simulink model "apilot2"  (Simulink 2.09)
settings: Solver=ode15s  StartTime=0.0  StopTime=140  MaxStep=4  RelTol=1e-04  AbsTol=1e-04
values from neighbouring files (symbols this model uses):
  CD = 0    [apinit.m]    (also in vorinit.m)
  gamgs = -3*pi/180    (= -0.0523598775598)    [apinit.m]    (also in ilsinit.m = -3)
  HRW = 0    [apinit.m]    (also in ilsinit.m)
  Sgs = 625/abs(gamgs)    [apinit.m]    (also in ilsinit.m)
  Sloc = 1.4*xloc    (= 2800)    [apinit.m]    (also in ilsinit.m)
  xgs = 300    [apinit.m]    (also in ilsinit.m)
  xloc = 2000    [apinit.m]    (also in ilsinit.m)
  ymod1A = [1 1 1 0 0]'    [apmode.m]
  ymod1S = [1 1 1 0 0]'    [apmode.m]
  ymod2A = [1 1 0 0 1]'    [apmode.m]
  ymod2S = [1 1 0 0 1]'    [apmode.m]
  yrefA = [0 Dpsir]'    [apmode.m]
  yrefS = [0 0 DHdotr]'    [apmode.m]
undefined symbols (not defined in the file or in its folder): Aail, Aelv, AM, Arud, Bail, Belv, Brud, Cail, Celv, Crud, Dail, Delv, Drud, GM1, sfunyst, uaero0, uprop0, xdot0, xfix, xinco
libraries: navlib1 x1, navlib2 x1
(part 1 of 2)
settings Model: SaveTime=off  SaveOutput=off  ConsistencyChecking=off  RTWTemplateMakefile=grt_vc.tmf

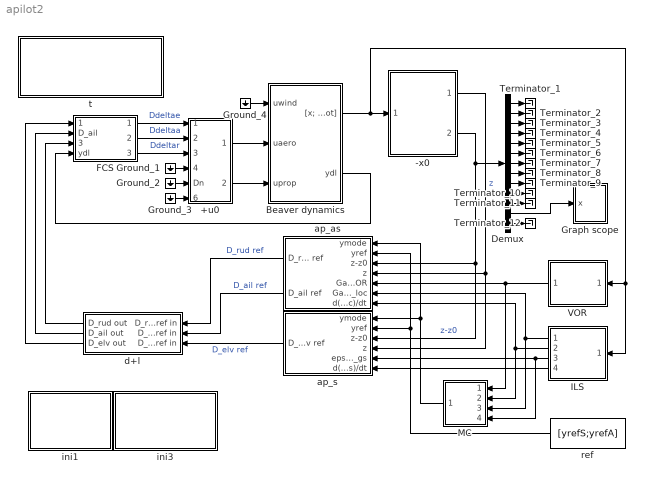
== system apilot2 ==
  +u0 : Subsystem
      mask Display: disp('Add\ninitial\ninputs')
  -x0 : Subsystem
      mask Display: disp('Subtract\ninitial con-\nditions\n\nNo sensors!')
  Beaver dynamics : Subsystem
  Demux : Demux  Outputs=13
  FCS : Subsystem
      mask Display: disp('Actuator &\ncable dy-\nnamics')
  Graph scope : Subsystem  mask(Storage scope.){npts=100, color='g-'}
      mask prompts: npts "Initial Time Range:"; color "Initial y-min:"
      mask help:
      | Storage scope using MATLAB graph window.
      | Enter plotting ranges and line type.
      mask init:
      | close all; ax = [0, @1, @2, @3];
      mask Help: Uses MATLAB's graph window.\nUse only one block per system.\nLine type must be in quotes.\nSee the M-file sfunyst.m.
      mask Display: plot(0,0,100,100,[83,76,63,52,42,38,28,16,11,84,11,11,11,90,90,11],[75,58,47,54,72,80,84,74,65,65,65,90,40,40,90,90])
  Ground_{1..4} (4 alike) : Ground
  ILS : Subsystem  Orientation=left
      mask Display: plot(0,0,100,100,[53,23,30,61,53],[45,60,64,49,45],[16,27,32,26],[48,40,43,47],[21,20,24,26,21],[44,55,56,47,44],[20,20,16],[50,50,48],[38,27,26,33],[52,46,48,55],[42,38,27],[50,47,46],[40,44,44,45,45,44,42],[48,44,42,42,44,44,50],[47,45,43],[55,58,58],[54,84,98,90,54],[36,21,56,58,36],[74,68],[34,29],[81,76],[43,38],[87,83],[49,45],[94,89],[57,52],[105,105],[0,0])
  MC : Subsystem  Orientation=left
      mask Display: disp('Mode\nCon-\ntroller')
  Terminator_{1..12} (12 alike) : Terminator
  VOR : Subsystem  Orientation=left
      mask Display: plot(0,0,100,100,[86,85,90,86,80,85,0],[16,80,20,16,20,80,62],[22,18,25,28,22,19],[36,32,29,33,36,45],[17,15,12,18,16,19],[37,37,34,32,44,46],[22,31,47,52,19,15,28,22],[36,44,39,44,55,50,45,38],[31,28],[44,45],[20,18,17],[31,30,32],[36,35,36,37,36,35,35,35,33,31,25],[41,38,33,32,30,30,32,33,37,35,34],[85,42],[80,50],[86,87,87,86,84,83,84,85],[83,81,78,76,76,79,82,83])
  ap_as : Subsystem  Orientation=left
      mask Display: disp('Asymmetrical\nautopilot\nmodes')
  ap_s : Subsystem  Orientation=left
      mask Display: disp('Symmetrical\nautopilot\nmodes')
  d+l : Subsystem  Orientation=left
      mask Display: disp('computational\ndelay & limiters')
  ini1 : Subsystem
      settings: OpenFcn=apinit
      mask Type: apinit
      mask Display: disp('1. Initialize\nsubsystems\n\nAPINIT')
  ini3 : Subsystem
      settings: OpenFcn=apmode
      mask Type: apmode
      mask Display: disp('2. Select mode &\nreference signals\n\nAPMODE')
  ref : Constant  Orientation=left  Value=[yrefS;yrefA]
      mask Display: disp('Reference\nsignals')
  t : Subsystem
      settings: OpenFcn=fdchelp apilot
      mask Display: disp('Apilot2 (no wind, turbu-\nlence, and sensor models,\nno ILS/VOR error signals)\nMarc Rauw, June 2000')
  wires:
  FCS/1(Ddeltae) -> +u0/1(Ddeltae)  "Ddeltae"
  FCS/2(Ddeltaa) -> +u0/2(Ddeltaa)  "Ddeltaa"
  FCS/3(Ddeltar) -> +u0/3(Ddeltar)  "Ddeltar"
  Ground_1/1 -> +u0/4(Ddeltaf)
  Ground_2/1 -> +u0/5(Dn)
  Ground_3/1 -> +u0/6(Dpz)
  Demux/12 -> Graph scope/1(x)
  ILS/2(d(Gamma_loc)/dt) -> ap_as/7(d(Gamma_loc)/dt), MC/2(d(Gamma_loc)/dt)
  -x0/2(z-z0 == [x-x0; Hdot-Hdot0]) -> Demux/1, ap_s/3(z-z0), ap_as/3(z-z0)  "z-z0"
  d+l/1(D_rud out) -> FCS/3(D_rud)
  d+l/2(D_ail out) -> FCS/2(D_ail)
  Beaver dynamics/1("[x; Hdot]") -> VOR/1("[x' ; Hdot]'"), ILS/1("[x' ;Hdot]'"), -x0/1("[x; Hdot]")
  Beaver dynamics/2(ydl) -> FCS/4(ydl)
  ap_as/2(D_ail ref) -> d+l/2(D_ail ref in)  "D_ail ref"
  ap_s/1(D_elv ref) -> d+l/3(D_elv ref in)  "D_elv ref"
  d+l/3(D_elv out) -> FCS/1(D_elv)
  ref/1 -> ap_s/2(yref), ap_as/2(yref)
  MC/1(ymode) -> ap_s/1(ymode), ap_as/1(ymode)
  +u0/1(uaero) -> Beaver dynamics/2(uaero)
  -x0/1("z == [x; Hdot] ") -> ap_as/4(z), ap_s/4(z)  "z"
  +u0/2(uprop) -> Beaver dynamics/3(uprop)
  VOR/1(Gamma_VOR) -> MC/1(Gamma_VOR), ap_as/5(Gamma_VOR)
  ILS/4(d(epsilon_gs)/dt) -> ap_s/6(d(epsilon_gs)/dt)
  ILS/1(Gamma_loc) -> MC/3(Gamma_loc), ap_as/6(Gamma_loc)
  ap_as/1(D_rud ref) -> d+l/1(D_rud ref in)  "D_rud ref"
  ILS/3(epsilon_gs) -> MC/4(epsilon_gs), ap_s/5(epsilon_gs)
  Demux/1 -> Terminator_1/1
  Demux/2 -> Terminator_2/1
  Demux/3 -> Terminator_3/1
  Demux/4 -> Terminator_4/1
  Demux/5 -> Terminator_5/1
  Demux/6 -> Terminator_6/1
  Demux/7 -> Terminator_7/1
  Demux/8 -> Terminator_8/1
  Demux/9 -> Terminator_9/1
  Demux/10 -> Terminator_10/1
  Demux/11 -> Terminator_11/1
  Demux/13 -> Terminator_12/1
  Ground_4/1 -> Beaver dynamics/1(uwind)

== system apilot2/+u0 ==
  note: Add initial inputs
  note: ENGINE INPUTS:
  note: AERODYNAMIC INPUTS:
  Ddeltae : Inport  Port=1  PortWidth=-1  SampleTime=-1
  Ddeltaa : Inport  Port=2  PortWidth=-1  SampleTime=-1
  Ddeltar : Inport  Port=3  PortWidth=-1  SampleTime=-1
  Ddeltaf : Inport  Port=4  PortWidth=-1  SampleTime=-1
  Dn : Inport  Port=5  PortWidth=-1  SampleTime=-1
  Dpz : Inport  Port=6  PortWidth=-1  SampleTime=-1
  Initial inputs for aeromod : Constant  Value=uaero0
  Initial inputs for engmod : Constant  Value=uprop0
  Mux1 : Mux  Inputs=4
  Mux2 : Mux  Inputs=2
  Sum : Sum  Inputs=++
  Sum1 : Sum  Inputs=++
  uaero : Outport  Port=1  InitialOutput=0
  uprop : Outport  Port=2  InitialOutput=0
  wires:
  Dpz/1 -> Mux2/2
  Dn/1 -> Mux2/1
  Initial inputs for engmod/1 -> Sum/2
  Mux2/1 -> Sum/1
  Sum/1 -> uprop/1
  Ddeltaa/1 -> Mux1/2
  Ddeltae/1 -> Mux1/1
  Ddeltar/1 -> Mux1/3
  Ddeltaf/1 -> Mux1/4
  Initial inputs for aeromod/1 -> Sum1/1
  Sum1/1 -> uaero/1
  Mux1/1 -> Sum1/2

== system apilot2/-x0 ==
  note: Subtract initial conditions
  "[x; Hdot]" : Inport  Port=1  PortWidth=-1  SampleTime=-1
  Initial condition : Constant  Value=[xinco; xdot0(12)]
  Sum : Sum  Inputs=+-
  "z == [x; Hdot] " : Outport  Port=1  InitialOutput=0
  z-z0 == [x-x0; Hdot-Hdot0] : Outport  Port=2  InitialOutput=0
  wires:
  "[x; Hdot]"/1 -> "z == [x; Hdot] "/1, Sum/1
  Initial condition/1 -> Sum/2
  Sum/1 -> z-z0 == [x-x0; Hdot-Hdot0]/1

== system apilot2/Beaver dynamics ==
  note: Beaver dynamics
      | and output equations
  uwind : Inport  Port=1  PortWidth=6  SampleTime=-1
  uaero : Inport  Port=2  PortWidth=4  SampleTime=-1
  uprop : Inport  Port=3  PortWidth=2  SampleTime=-1
  0 : Subsystem
      settings: OpenFcn=fdchelp level1
      mask Display: disp('Subsystem equivalent of\nthe S-function BEAVER\nM.O. Rauw, October 1997')
  AC : Subsystem
  Clock : Clock
  Demux1 : Demux  Outputs=[11 1]
  Mux : Mux  Inputs=[12 1]
  Mux_in : Mux  Orientation=up  Inputs=[4 2 6]
      settings: OpenFcn=fdchelp inputs
      mask Display: disp('Mux\nclick\n2x for\ninfo!')
  Mux_out : Mux  Orientation=up  Inputs=[12 12 3 3 3 4 2 6 6 6 6 6 3 3 5 3 3 3]
      settings: OpenFcn=fdchelp outputs
      mask Display: disp('Mux\n\nDouble-click for info!')
  Terminator_1 : Terminator
  To Workspace : ToWorkspace  VariableName=Out  SampleTime=0
      settings: Orientation=up  Buffer=5000
  "To Workspace " : ToWorkspace  VariableName=In  SampleTime=0
      settings: Orientation=up  Buffer=5000
  "To Workspace  " : ToWorkspace  VariableName=time  SampleTime=0
      settings: Buffer=5000
  "[x; Hdot]" : Outport  Port=1  InitialOutput=0
  ydl : Outport  Port=2  InitialOutput=0
  wires:
  Mux/1 -> "[x; Hdot]"/1
  Demux1/2 -> Mux/2  "Hdot"
  Demux1/1 -> Terminator_1/1
  uaero/1 -> Mux_in/1, AC/1(uaero)
  uprop/1 -> Mux_in/2, AC/2(uprop)
  uwind/1 -> Mux_in/3, AC/3(" uwind")
  AC/18(yad3) -> Mux_out/18
  AC/17(yad2) -> Mux_out/17
  AC/4(yuvw) -> Mux_out/4
  AC/1(x) -> Mux_out/1, Mux/1  "x"
  AC/3(ybvel) -> Mux_out/3
  AC/16(yad1) -> Mux_out/16
  AC/5(ydl) -> Mux_out/5, ydl/1
  AC/6(yfp) -> Mux_out/6
  AC/8(yacc) -> Mux_out/8
  AC/9(Caero) -> Mux_out/9
  AC/10(Cprop) -> Mux_out/10
  AC/11(FMaero) -> Mux_out/11
  AC/12(FMprop) -> Mux_out/12
  AC/13(Fgrav) -> Mux_out/13
  AC/14(Fwind) -> Mux_out/14
  AC/15(yatm) -> Mux_out/15
  AC/2(xdot) -> Demux1/1, Mux_out/2  "xdot"
  Clock/1 -> "To Workspace  "/1
  Mux_out/1 -> To Workspace/1
  Mux_in/1 -> "To Workspace "/1
  AC/7(ypow) -> Mux_out/7

== system apilot2/FCS ==
  note: Actuators
      | + cables:
  D_elv : Inport  Port=1  PortWidth=-1  SampleTime=-1
  D_ail : Inport  Port=2  PortWidth=-1  SampleTime=-1
  D_rud : Inport  Port=3  PortWidth=-1  SampleTime=-1
  ydl : Inport  Port=4  PortWidth=-1  SampleTime=-1
  Demux1 : Demux  Outputs=3
  Mux1 : Mux  Inputs=2
  Mux2 : Mux  Inputs=2
  Mux3 : Mux  Inputs=2
  ailerons : StateSpace  A=Aail  B=Bail  C=Cail*2  D=Dail  X0=0
  elevator : StateSpace  A=Aelv  B=Belv  C=Celv  D=Delv  X0=0
  rudder : StateSpace  A=Arud  B=Brud  C=Crud  D=Drud  X0=0
  t : Subsystem
      settings: OpenFcn=fdchelp actuatr
      mask Display: disp('Actuator & cable dynamics\nMarc Rauw, October 1997')
  Ddeltae : Outport  Port=1  InitialOutput=0
  Ddeltaa : Outport  Port=2  InitialOutput=0
  Ddeltar : Outport  Port=3  InitialOutput=0
  wires:
  Demux1/2 -> Mux1/2
  Demux1/1 -> Mux2/2
  Demux1/3 -> Mux3/2
  Mux1/1 -> elevator/1
  Mux2/1 -> ailerons/1
  Mux3/1 -> rudder/1
  elevator/1 -> Ddeltae/1
  ailerons/1 -> Ddeltaa/1
  ydl/1 -> Demux1/1
  rudder/1 -> Ddeltar/1
  D_elv/1 -> Mux1/1
  D_ail/1 -> Mux2/1
  D_rud/1 -> Mux3/1

== system apilot2/Graph scope ==
  x : Inport  Port=1  PortWidth=-1  SampleTime=-1
  "S-function M-file which plots lines " : S-Function  LoadFcn=sfunyst([],[],[],'LoadBlock')  FunctionName=sfunyst  Parameters=ax, color, npts
      settings: CopyFcn=sfunyst([],[],[],'CopyBlock')  DeleteFcn=sfunyst([],[],[],'DeleteBlock')
  wires:
  x/1 -> "S-function M-file which plots lines "/1

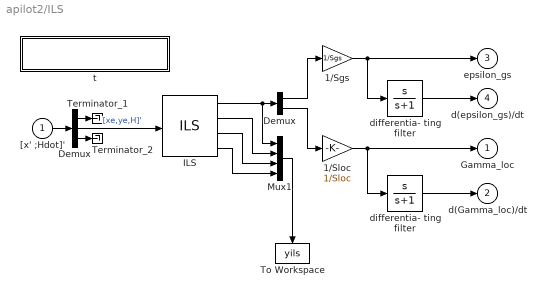
== system apilot2/ILS ==
  "[x' ;Hdot]'" : Inport  Port=1  PortWidth=-1  SampleTime=-1
  1/Sgs : Gain  Gain=1/Sgs
  1/Sloc : Gain  Gain=1/Sloc
  Demux : Demux  Outputs=2
  "Demux " : Demux  Outputs=[9 3 1]
  ILS : navlib1/ILS  RWpos=[20000,-100,0]  MaskParam1=0  MaskParam3=2200  MaskParam4=300  MaskParam5=100  MaskParam6=3
  Mux1 : Mux  Inputs=[2 2 6 2]
  Terminator_1 : Terminator
  Terminator_2 : Terminator
  To Workspace : ToWorkspace  VariableName=yils  SampleTime=0
      settings: Orientation=down  Buffer=5000
  differentia- ting filter : TransferFcn  Numerator=[1 0]  Denominator=[1 1]
  "differentia- ting filter " : TransferFcn  Numerator=[1 0]  Denominator=[1 1]
  t : Subsystem
      mask Display: disp('ILS signals (no error signals)\nMarc Rauw, January 1998')
  Gamma_loc : Outport  Port=1  InitialOutput=0
  d(Gamma_loc)/dt : Outport  Port=2  InitialOutput=0
  epsilon_gs : Outport  Port=3  InitialOutput=0
  d(epsilon_gs)/dt : Outport  Port=4  InitialOutput=0
  wires:
  Demux/2 -> 1/Sloc/1
  Demux/1 -> 1/Sgs/1
  ILS/2 -> Mux1/2
  ILS/3 -> Mux1/3
  ILS/1 -> Mux1/1, Demux/1
  ILS/4 -> Mux1/4
  Mux1/1 -> To Workspace/1
  1/Sloc/1 -> differentia- ting filter/1, Gamma_loc/1
  1/Sgs/1 -> "differentia- ting filter "/1, epsilon_gs/1
  differentia- ting filter/1 -> d(Gamma_loc)/dt/1
  "differentia- ting filter "/1 -> d(epsilon_gs)/dt/1
  "Demux "/2 -> ILS/1  "[xe,ye,H]'"
  "Demux "/1 -> Terminator_1/1
  "Demux "/3 -> Terminator_2/1
  "[x' ;Hdot]'"/1 -> "Demux "/1

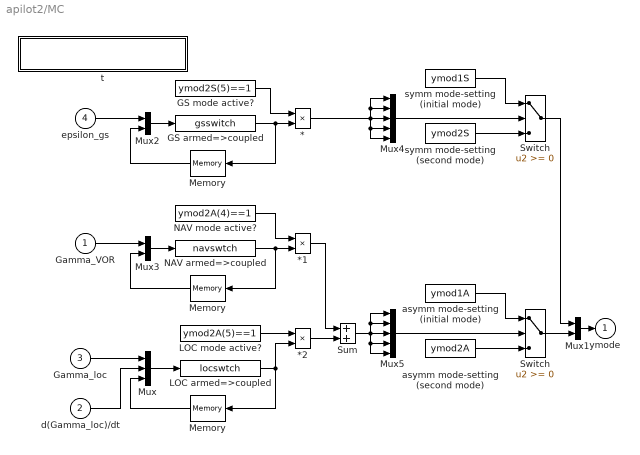
== system apilot2/MC ==
  Gamma_VOR : Inport  Port=1  PortWidth=-1  SampleTime=-1
  d(Gamma_loc)/dt : Inport  Port=2  PortWidth=-1  SampleTime=-1
  Gamma_loc : Inport  Port=3  PortWidth=-1  SampleTime=-1
  epsilon_gs : Inport  Port=4  PortWidth=-1  SampleTime=-1
  " Memory" : Memory  Orientation=left  X0=0  InheritSampleTime=off
  * : Product  Inputs=2
  *1 : Product  Inputs=2
  *2 : Product  Inputs=2
  GS armed=>coupled : MATLABFcn  MATLABFcn=gsswitch  OutputWidth=1
      mask Display: disp('gsswitch.m')
  GS mode active? : Constant  Value=ymod2S(5)==1
  LOC armed=>coupled : MATLABFcn  MATLABFcn=locswtch  OutputWidth=1
      mask Display: disp('locswtch.m')
  LOC mode active? : Constant  Value=ymod2A(5)==1
  Memory : Memory  Orientation=left  X0=1  InheritSampleTime=off
  "Memory " : Memory  Orientation=left  X0=0  InheritSampleTime=off
  Mux : Mux  Inputs=3
  Mux1 : Mux  Inputs=[5 5]
  Mux2 : Mux  Inputs=2
  Mux3 : Mux  Inputs=2
  Mux4 : Mux  Inputs=5
  Mux5 : Mux  Inputs=5
  NAV armed=>coupled : MATLABFcn  MATLABFcn=navswtch  OutputWidth=1
      mask Display: disp('navswtch.m')
  NAV mode active? : Constant  Value=ymod2A(4)==1
  Sum : Sum  Inputs=++
  Switch : Switch  Threshold=0
  "Switch " : Switch  Threshold=0
  asymm mode-setting (initial mode) : Constant  Value=ymod1A
  asymm mode-setting (second mode) : Constant  Value=ymod2A
  symm mode-setting (initial mode) : Constant  Value=ymod1S
  symm mode-setting (second mode) : Constant  Value=ymod2S
  t : Subsystem
      settings: OpenFcn=fdchelp modectrl
      mask Display: disp('Mode-controller\nM.O. Rauw, October 1997')
  ymode : Outport  Port=1  InitialOutput=0
  wires:
  Mux/1 -> LOC armed=>coupled/1
  Gamma_loc/1 -> Mux/1
  Mux2/1 -> GS armed=>coupled/1
  epsilon_gs/1 -> Mux2/1
  Mux3/1 -> NAV armed=>coupled/1
  Gamma_VOR/1 -> Mux3/1
  d(Gamma_loc)/dt/1 -> Mux/2
  Mux4/1 -> Switch/2
  Mux5/1 -> "Switch "/2
  GS armed=>coupled/1 -> Memory/1, */2
  "Switch "/1 -> Mux1/2
  Mux1/1 -> ymode/1
  GS mode active?/1 -> */1
  NAV armed=>coupled/1 -> "Memory "/1, *1/2
  NAV mode active?/1 -> *1/1
  LOC mode active?/1 -> *2/1
  *2/1 -> Sum/2
  asymm mode-setting (second mode)/1 -> "Switch "/3
  LOC armed=>coupled/1 -> *2/2, " Memory"/1
  */1 -> Mux4/3, Mux4/1, Mux4/2, Mux4/5, Mux4/4
  Memory/1 -> Mux2/2
  "Memory "/1 -> Mux3/2
  " Memory"/1 -> Mux/3
  symm mode-setting (second mode)/1 -> Switch/3
  Switch/1 -> Mux1/1
  Sum/1 -> Mux5/3, Mux5/5, Mux5/4, Mux5/1, Mux5/2
  *1/1 -> Sum/1
  symm mode-setting (initial mode)/1 -> Switch/1
  asymm mode-setting (initial mode)/1 -> "Switch "/1

== system apilot2/VOR ==
  "[x' ; Hdot]'" : Inport  Port=1  PortWidth=-1  SampleTime=-1
  Demux : Demux  Outputs=[6 1 2 3 1]
  Mux1 : Mux  Inputs=[1 1 2 1]
  Terminator_1 : Terminator
  Terminator_2 : Terminator
  Terminator_3 : Terminator
  To Workspace : ToWorkspace  VariableName=yvor  SampleTime=0
      settings: Buffer=5000
  VOR : navlib2/VOR  xVOR=xVOR  yVOR=yVOR  HVOR=HVOR  MaskParam4=CD
  t : Subsystem
      mask Display: disp('VOR signals (no error signals)\nMarc Rauw, January 1998')
  Gamma_VOR : Outport  Port=1  InitialOutput=0
  wires:
  VOR/1 -> Mux1/1, Gamma_VOR/1
  Mux1/1 -> To Workspace/1
  VOR/2 -> Mux1/2
  VOR/3 -> Mux1/3
  VOR/4 -> Mux1/4
  Demux/4 -> VOR/1  "[xe,ye,H]'"
  Demux/2 -> VOR/2  "psi"
  "[x' ; Hdot]'"/1 -> Demux/1
  Demux/1 -> Terminator_1/1
  Demux/3 -> Terminator_2/1
  Demux/5 -> Terminator_3/1

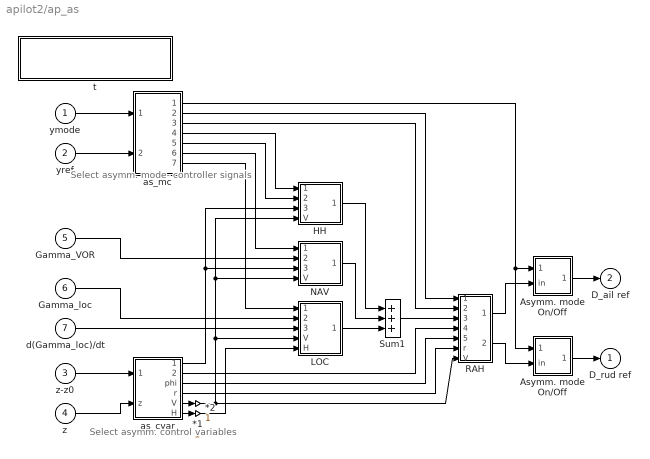
== system apilot2/ap_as ==
  note: Select asymm. mode-
      | controller signals
  note: Select asymm.
      | control variables
  ymode : Inport  Port=1  PortWidth=-1  SampleTime=-1
  yref : Inport  Port=2  PortWidth=-1  SampleTime=-1
  z-z0 : Inport  Port=3  PortWidth=-1  SampleTime=-1
  z : Inport  Port=4  PortWidth=-1  SampleTime=-1
  Gamma_VOR : Inport  Port=5  PortWidth=-1  SampleTime=-1
  Gamma_loc : Inport  Port=6  PortWidth=-1  SampleTime=-1
  d(Gamma_loc)/dt : Inport  Port=7  PortWidth=-1  SampleTime=-1
  *1 : Gain  Gain=1
  *2 : Gain  Gain=1
  Asymm. mode On/Off : Subsystem
      mask Type: On/off switch
      mask Description:
      | If input(1) = 1
      |      output = input(2)
      |  else if input(1) = 0
      |      output = 0
      mask Help: On/off switch.
      mask Display: plot(0,0,100,100,[31,31,32,34,34,32,31,31,0],[50,48,47,48,51,53,51,50,50],[100,75,51],[50,50,97]);disp('?')
  "Asymm. mode On/Off " : Subsystem
      mask Type: On/off switch
      mask Description:
      | If input(1) = 1
      |      output = input(2)
      |  else if input(1) = 0
      |      output = 0
      mask Help: On/off switch.
      mask Display: plot(0,0,100,100,[31,31,32,34,34,32,31,31,0],[50,48,47,48,51,53,51,50,50],[100,75,51],[50,50,97]);disp('?')
  HH : Subsystem
  LOC : Subsystem
  NAV : Subsystem
  RAH : Subsystem
  Sum1 : Sum  Inputs=+++
  as_cvar : Subsystem
  as_mc : Subsystem
  t : Subsystem
      settings: OpenFcn=fdchelp ap_asymm
      mask Display: disp('Asymm. autopilot modes\nMarc Rauw, October 1997')
  D_rud ref : Outport  Port=1  InitialOutput=0
  D_ail ref : Outport  Port=2  InitialOutput=0
  wires:
  z/1 -> as_cvar/2(z)
  d(Gamma_loc)/dt/1 -> LOC/3(d(Gamma_loc)/dt)
  Gamma_loc/1 -> LOC/2(Gamma_loc)
  Gamma_VOR/1 -> NAV/2(Gamma_VOR)
  as_mc/5(Dpsir (HH)) -> HH/2(Dpsir (HH))
  Sum1/1 -> RAH/3(Dphir (out. loop))
  *2/1 -> LOC/5(H)
  *1/1 -> RAH/7(V), LOC/4(V), HH/4(V), NAV/4(V)
  as_cvar/6(H) -> *2/1
  as_mc/7(LOC coupled?) -> LOC/1(LOC coupled?)
  as_mc/6(NAV?) -> NAV/1(NAV?)
  as_mc/4(HH?) -> HH/1(HH?)
  as_mc/3(Dphir (RAH)) -> RAH/2(Dphir (RAH))
  as_mc/2(asymm. out. loop?) -> RAH/1(Asymm out. loop?)
  as_cvar/2(phi-phi0) -> RAH/4(phi-phi0)
  as_cvar/3(phi) -> RAH/5(phi)
  as_cvar/4(r) -> RAH/6(r)
  as_cvar/5(V) -> *1/1
  LOC/1(Dphir (LOC)) -> Sum1/3
  NAV/1(Dphir (NAV)) -> Sum1/2
  ymode/1 -> as_mc/1(ymode)
  yref/1 -> as_mc/2(yref)
  "Asymm. mode On/Off "/1(out) -> D_ail ref/1
  Asymm. mode On/Off/1(out) -> D_rud ref/1
  z-z0/1 -> as_cvar/1(z-z0)
  as_cvar/1(psi-psi0) -> HH/3(psi-psi0), NAV/3(psi-psi0)
  RAH/1(D_ail ref) -> "Asymm. mode On/Off "/2(in)
  RAH/2(D_rud ref) -> Asymm. mode On/Off/2(in)
  HH/1(Dphir (HH)) -> Sum1/1
  as_mc/1(asymm. mode?) -> "Asymm. mode On/Off "/1(crit), Asymm. mode On/Off/1(crit)

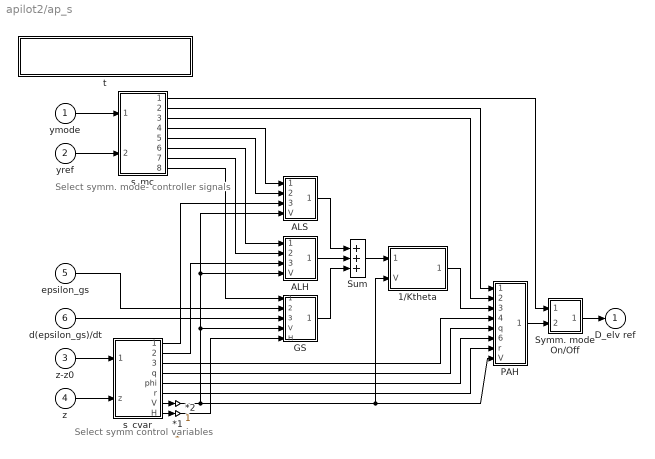
== system apilot2/ap_s ==
  note: Select symm. mode-
      | controller signals
  note: Select symm
      | control variables
  ymode : Inport  Port=1  PortWidth=-1  SampleTime=-1
  yref : Inport  Port=2  PortWidth=-1  SampleTime=-1
  z-z0 : Inport  Port=3  PortWidth=-1  SampleTime=-1
  z : Inport  Port=4  PortWidth=-1  SampleTime=-1
  epsilon_gs : Inport  Port=5  PortWidth=-1  SampleTime=-1
  d(epsilon_gs)/dt : Inport  Port=6  PortWidth=-1  SampleTime=-1
  *1 : Gain  Gain=1
  *2 : Gain  Gain=1
  1/Ktheta : Subsystem
      mask Display: plot(0,0,100,100,[0,100,0],[0,50,100]);disp('K(u1)      ')
  ALH : Subsystem
  ALS : Subsystem
  GS : Subsystem
  PAH : Subsystem
  Sum : Sum  Inputs=+++
  Symm. mode On/Off : Subsystem
      mask Type: On/off switch
      mask Description:
      | If input(1) = 1
      |      output = input(2)
      |  else if input(1) = 0
      |      output = 0
      mask Help: On/off switch. \nIf input(1) = 1, the output equals input(1). \nIf input(1) = 0, the output is zero.
      mask Display: plot(0,0,100,100,[31,31,32,34,34,32,31,31,0],[50,48,47,48,51,53,51,50,50],[100,75,51],[50,50,97]);disp('?')
  s_cvar : Subsystem
  s_mc : Subsystem
  t : Subsystem
      settings: OpenFcn=fdchelp ap_symm
      mask Display: disp('Symm. autopilot modes\nMarc Rauw, October 1997')
  D_elv ref : Outport  Port=1  InitialOutput=0
  wires:
  epsilon_gs/1 -> GS/2(epsilon_gs)
  d(epsilon_gs)/dt/1 -> GS/3(d(epsilon_gs)/dt)
  *1/1 -> PAH/8(V), 1/Ktheta/2(V), ALS/4(V), ALH/4(V), GS/4(V)
  1/Ktheta/1(y = K*u) -> PAH/3(Dthetar (out. loop))
  Sum/1 -> 1/Ktheta/1(input u)
  GS/1(Dthetar (GS)) -> Sum/3
  s_mc/1(symm mode?) -> Symm. mode On/Off/1(crit)
  Symm. mode On/Off/1(out) -> D_elv ref/1
  PAH/1(D_elv ref) -> Symm. mode On/Off/2(in)
  ALS/1(Dthetar (ALS)) -> Sum/1
  ALH/1(Dthetar (ALH)) -> Sum/2
  s_cvar/1(Hdot-Hdot0) -> ALS/3(Hdot-Hdot0)
  s_cvar/2(H-H0) -> ALH/3(H-H0)
  s_cvar/3(theta-theta0) -> PAH/4(theta-theta0)
  s_cvar/4(q) -> PAH/5(q)
  s_cvar/5(phi) -> PAH/6(phi)
  s_cvar/6(r) -> PAH/7(r)
  s_cvar/7(V) -> *1/1
  z-z0/1 -> s_cvar/1(z-z0)
  z/1 -> s_cvar/2(z)
  s_mc/2(symm. outer loop?) -> PAH/1(Symm out. loop?)
  s_mc/3(Dthetar (PAH)) -> PAH/2(Dthetar (PAH/GA))
  s_mc/4(ALS?) -> ALS/1(ALS?)
  s_mc/5(DHdot r (ALS)) -> ALS/2(DHdot r (ALS))
  s_mc/6(ALH?) -> ALH/1(ALH?)
  s_mc/7(DHr (ALH)) -> ALH/2(DHr (ALH))
  ymode/1 -> s_mc/1(ymode)
  yref/1 -> s_mc/2(yref)
  s_cvar/8(H) -> *2/1
  *2/1 -> GS/5(H)
  s_mc/8(GS coupled?) -> GS/1(GS coupled?)

== system apilot2/d+l ==
  D_rud ref in : Inport  Port=1  PortWidth=-1  SampleTime=-1
  D_ail ref in : Inport  Port=2  PortWidth=-1  SampleTime=-1
  D_elv ref in : Inport  Port=3  PortWidth=-1  SampleTime=-1
  " +/- 10 V " : Saturate  UpperLimit=10 * (pi/180)  LowerLimit=-10 * (pi/180)
  " delay" : TransportDelay  DelayTime=0.03  InitialInput=0  BufferSize=1024
  +/- 10 V : Saturate  UpperLimit=10 * (pi/180)  LowerLimit=-10 * (pi/180)
  "+/- 10 V " : Saturate  UpperLimit=10 * (pi/180)  LowerLimit=-10 * (pi/180)
  delay : TransportDelay  DelayTime=0.03  InitialInput=0  BufferSize=1024
  "delay " : TransportDelay  DelayTime=0.03  InitialInput=0  BufferSize=1024
  t : Subsystem
      settings: OpenFcn=fdchelp delaylim
      mask Display: disp('Computational delay and\ninput limiters (+- 10 Volt)\nMarc Rauw, October 1997')
  D_rud out : Outport  Port=1  InitialOutput=0
  D_ail out : Outport  Port=2  InitialOutput=0
  D_elv out : Outport  Port=3  InitialOutput=0
  wires:
  D_rud ref in/1 -> delay/1
  delay/1 -> +/- 10 V/1
  D_elv ref in/1 -> " delay"/1
  " +/- 10 V "/1 -> D_elv out/1
  D_ail ref in/1 -> "delay "/1
  "+/- 10 V "/1 -> D_ail out/1
  +/- 10 V/1 -> D_rud out/1
  " delay"/1 -> " +/- 10 V "/1
  "delay "/1 -> "+/- 10 V "/1

== system apilot2/ini1 ==

== system apilot2/ini3 ==

== system apilot2/t ==

== system apilot2/Beaver dynamics/0 ==

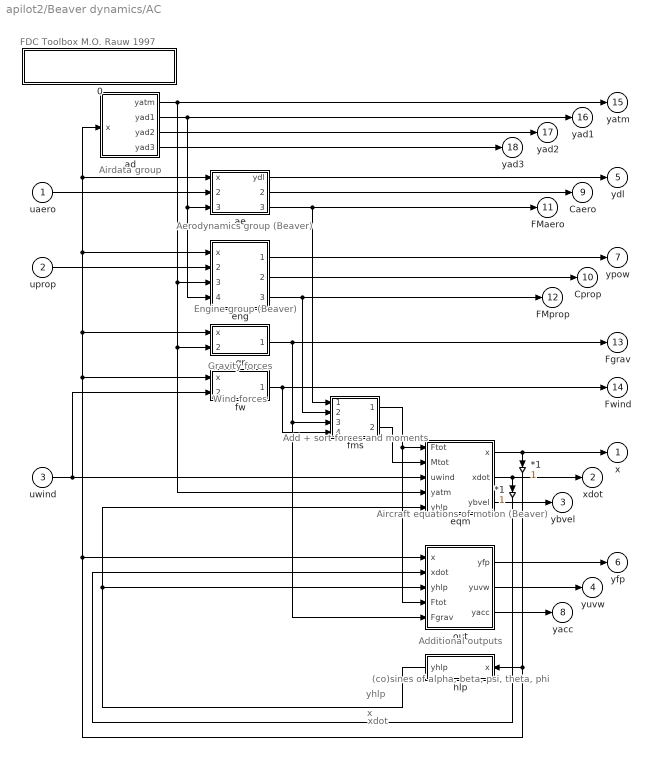
== system apilot2/Beaver dynamics/AC ==
  note: Airdata group
  note: Add + sort
      | forces and
      | moments
  note: (co)sines of
      | alpha, beta,
      | psi, theta, phi
  note: Aerodynamics
      | group (Beaver)
  note: Engine group (Beaver)
  note: Gravity forces
  note: Wind forces
  note: Aircraft equations
      | of motion (Beaver)
  note: Additional outputs
  note: yhlp
  note: x
  note: xdot
  note: FDC Toolbox
      |  M.O. Rauw 1997
  uaero : Inport  Port=1  PortWidth=-1  SampleTime=-1
  uprop : Inport  Port=2  PortWidth=-1  SampleTime=-1
  " uwind" : Inport  Port=3  PortWidth=-1  SampleTime=-1
  " *1" : Gain  Orientation=down  Gain=1
  *1 : Gain  Orientation=down  Gain=1
  0 : Subsystem
      settings: OpenFcn=fdchelp level2
      mask Display: disp('BEAVER, level 2 (main level)\nM.O. Rauw')
  ad : Subsystem
  ae : Subsystem
  eng : Subsystem
  eqm : Subsystem
  fms : Subsystem
      mask Type: FMsort
      mask Description: Forces and Moments sorting block
      mask Help: eval('fdchelp fmsort')
      mask Display: disp('FMsort')
  fw : Subsystem  mask(fwind){m=GM1(10)}
      mask prompts: m "Mass of the aircraft [kg]:"
      mask help: Forces due to non-steady atmosphere.
      mask Help: eval('fdchelp fwind')
      mask Display: disp('Fwind')
  gr : Subsystem  mask(Gravity){m=GM1(10)}
      mask prompts: m "Mass of the aircraft [kg]:"
      mask help: Gravity forces.
      mask Help: eval('fdchelp gravity')
      mask Display: disp('Gravity')
  hlp : Subsystem  Orientation=left
      mask Type: Hlpfcn
      mask Description: Help sines and cosines
      mask Help: eval('fdchelp hlpfcn')
      mask Display: disp('hlpfcn')
  out : Subsystem
  x : Outport  Port=1  InitialOutput=0
  xdot : Outport  Port=2  InitialOutput=0
  ybvel : Outport  Port=3  InitialOutput=0
  yuvw : Outport  Port=4  InitialOutput=0
  ydl : Outport  Port=5  InitialOutput=0
  yfp : Outport  Port=6  InitialOutput=0
  ypow : Outport  Port=7  InitialOutput=0
  yacc : Outport  Port=8  InitialOutput=0
  Caero : Outport  Port=9  InitialOutput=0
  Cprop : Outport  Port=10  InitialOutput=0
  FMaero : Outport  Port=11  InitialOutput=0
  FMprop : Outport  Port=12  InitialOutput=0
  Fgrav : Outport  Port=13  InitialOutput=0
  Fwind : Outport  Port=14  InitialOutput=0
  yatm : Outport  Port=15  InitialOutput=0
  yad1 : Outport  Port=16  InitialOutput=0
  yad2 : Outport  Port=17  InitialOutput=0
  yad3 : Outport  Port=18  InitialOutput=0
  wires:
  fms/2(Mtot) -> eqm/2(Mtot)
  fms/1(Ftot) -> eqm/1(Ftot), out/4(Ftot)
  eqm/1(x) -> " *1"/1, x/1
  eqm/2(xdot) -> *1/1, xdot/1
  " *1"/1 -> ad/1(x), ae/1(x), eng/1(x), gr/1(x), fw/1(x), out/1(x), hlp/1(x)
  gr/1(Fgrav) -> out/5(Fgrav), fms/3(Fgrav), Fgrav/1
  *1/1 -> out/2(xdot)
  " uwind"/1 -> fw/2(uwind), eqm/3(uwind)
  hlp/1(yhlp) -> out/3(yhlp), eqm/5(yhlp)
  ae/3(FMaero) -> fms/1(FMaero), FMaero/1
  eng/3(FMprop) -> fms/2(FMprop), FMprop/1
  fw/1(Fwind) -> fms/4(Fwind), Fwind/1
  out/3(yacc) -> yacc/1
  ad/1(yatm) -> gr/2(yatm), eqm/4(yatm), eng/3(yatm), yatm/1
  ad/3(yad2) -> yad2/1
  ad/2(yad1) -> yad1/1, ae/3(yad1), eng/4(yad1)
  out/1(yfp) -> yfp/1
  eqm/3(ybvel) -> ybvel/1
  eng/2(Cprop) -> Cprop/1
  eng/1(ypow) -> ypow/1
  ae/2(Caero) -> Caero/1
  ae/1(ydl) -> ydl/1
  ad/4(yad3) -> yad3/1
  uaero/1 -> ae/2(uaero)
  uprop/1 -> eng/2(uprop)
  out/2(yuvw) -> yuvw/1

== system apilot2/FCS/t ==

== system apilot2/ILS/t ==

== system apilot2/MC/t ==

== system apilot2/VOR/t ==

== system apilot2/ap_as/Asymm. mode On/Off ==
  crit : Inport  Port=1  PortWidth=-1  SampleTime=-1
  in : Inport  Port=2  PortWidth=-1  SampleTime=-1
  Sum : Sum  Inputs=+-
  Switch : Switch  Threshold=0
  const. : Constant  Value=0.5
  const.1 : Constant  Value=0
  out : Outport  Port=1  InitialOutput=0
  wires:
  const./1 -> Sum/2
  in/1 -> Switch/1
  Switch/1 -> out/1
  Sum/1 -> Switch/2
  const.1/1 -> Switch/3
  crit/1 -> Sum/1

== system apilot2/ap_as/Asymm. mode On/Off  ==
  crit : Inport  Port=1  PortWidth=-1  SampleTime=-1
  in : Inport  Port=2  PortWidth=-1  SampleTime=-1
  Sum : Sum  Inputs=+-
  Switch : Switch  Threshold=0
  const. : Constant  Value=0.5
  const.1 : Constant  Value=0
  out : Outport  Port=1  InitialOutput=0
  wires:
  crit/1 -> Sum/1
  const.1/1 -> Switch/3
  Sum/1 -> Switch/2
  Switch/1 -> out/1
  in/1 -> Switch/1
  const./1 -> Sum/2

== system apilot2/ap_as/HH ==
  note: Heading Hold / Heading Select mode
  HH? : Inport  Port=1  PortWidth=-1  SampleTime=-1
  Dpsir (HH) : Inport  Port=2  PortWidth=-1  SampleTime=-1
  psi-psi0 : Inport  Port=3  PortWidth=-1  SampleTime=-1
  V : Inport  Port=4  PortWidth=-1  SampleTime=-1
  Kpsi : Subsystem
      mask Display: plot(0,0,100,100,[0,100,0],[0,50,100]);disp('K(u1)      ')
  On/Off : Subsystem
      mask Type: On/off switch
      mask Description:
      | If input(1) = 1
      |      output = input(2)
      |  else if input(1) = 0
      |      output = 0
      mask Help: On/off switch.
      mask Display: plot(0,0,100,100,[31,31,32,34,34,32,31,31,0],[50,48,47,48,51,53,51,50,50],[100,75,51],[50,50,97]);disp('?')
  Sum : Sum  Inputs=+-
  Dphir (HH) : Outport  Port=1  InitialOutput=0
  wires:
  V/1 -> Kpsi/1(V)
  HH?/1 -> On/Off/1(crit)
  Dpsir (HH)/1 -> Sum/1
  psi-psi0/1 -> Sum/2
  Kpsi/1(y = K*u) -> On/Off/2(in)
  Sum/1 -> Kpsi/2(input u)
  On/Off/1(out) -> Dphir (HH)/1

== system apilot2/ap_as/LOC ==
  note: Localizer coupled mode
  LOC coupled? : Inport  Port=1  PortWidth=-1  SampleTime=-1
  Gamma_loc : Inport  Port=2  PortWidth=-1  SampleTime=-1
  d(Gamma_loc)/dt : Inport  Port=3  PortWidth=-1  SampleTime=-1
  V : Inport  Port=4  PortWidth=-1  SampleTime=-1
  H : Inport  Port=5  PortWidth=-1  SampleTime=-1
  KGam_LOC : Subsystem
      mask Display: plot(0,0,100,100,[0,100,0],[0,50,100]);disp('K(u1)       ')
  Kv : Gain  Gain=10
  On/Off : Subsystem
      mask Type: On/off switch
      mask Description:
      | If input(1) = 1
      |      output = input(2)
      |  else if input(1) = 0
      |      output = 0
      mask Help: On/off switch.
      mask Display: plot(0,0,100,100,[31,31,32,34,34,32,31,31,0],[50,48,47,48,51,53,51,50,50],[100,75,51],[50,50,97]);disp('?')
  Rloc approximation : Fcn  Expr=(u[1]-HRW)/sin(abs(gamgs*pi/180)) + xloc
  Sum : Sum  Inputs=++
  prod : Product  Inputs=2
  Dphir (LOC) : Outport  Port=1  InitialOutput=0
  wires:
  V/1 -> KGam_LOC/1(V)
  Gamma_loc/1 -> Sum/1
  Kv/1 -> Sum/2
  d(Gamma_loc)/dt/1 -> Kv/1
  Sum/1 -> prod/1
  H/1 -> Rloc approximation/1
  prod/1 -> KGam_LOC/2(input u)
  KGam_LOC/1(y = K*u) -> On/Off/2(in)
  LOC coupled?/1 -> On/Off/1(crit)
  On/Off/1(out) -> Dphir (LOC)/1
  Rloc approximation/1 -> prod/2

== system apilot2/ap_as/NAV ==
  note: VOR navigation mode
  NAV? : Inport  Port=1  PortWidth=-1  SampleTime=-1
  Gamma_VOR : Inport  Port=2  PortWidth=-1  SampleTime=-1
  psi-psi0 : Inport  Port=3  PortWidth=-1  SampleTime=-1
  V : Inport  Port=4  PortWidth=-1  SampleTime=-1
  Dpsir (NAV) : Constant  Value=CD-xinco(7)
  KGam_VOR : Subsystem
      mask Display: plot(0,0,100,100,[0,100,0],[0,50,100]);disp('K(u1)     ')
  Kpsi : Subsystem
      mask Display: plot(0,0,100,100,[0,100,0],[0,50,100]);disp('K(u1)      ')
  Low-pass filter : TransferFcn  Numerator=[1]  Denominator=[1 1]
  On/Off : Subsystem
      mask Type: On/off switch
      mask Description:
      | If input(1) = 1
      |      output = input(2)
      |  else if input(1) = 0
      |      output = 0
      mask Help: On/off switch.
      mask Display: plot(0,0,100,100,[31,31,32,34,34,32,31,31,0],[50,48,47,48,51,53,51,50,50],[100,75,51],[50,50,97]);disp('?')
  Sum : Sum  Inputs=++
  Sum1 : Sum  Inputs=+-
  Washout filter (includes forward loop below) : TransferFcn  Numerator=[15 0]  Denominator=[15 1]
  Dphir (NAV) : Outport  Port=1  InitialOutput=0
  wires:
  V/1 -> Kpsi/1(V), KGam_VOR/1(V)
  psi-psi0/1 -> Sum1/2
  NAV?/1 -> On/Off/1(crit)
  On/Off/1(out) -> Dphir (NAV)/1
  Sum/1 -> On/Off/2(in)
  Washout filter (includes forward loop below)/1 -> Sum/2
  Kpsi/1(y = K*u) -> Washout filter (includes forward loop below)/1
  Low-pass filter/1 -> Sum/1
  KGam_VOR/1(y = K*u) -> Low-pass filter/1
  Gamma_VOR/1 -> KGam_VOR/2(input u)
  Sum1/1 -> Kpsi/2(input u)
  Dpsir (NAV)/1 -> Sum1/1

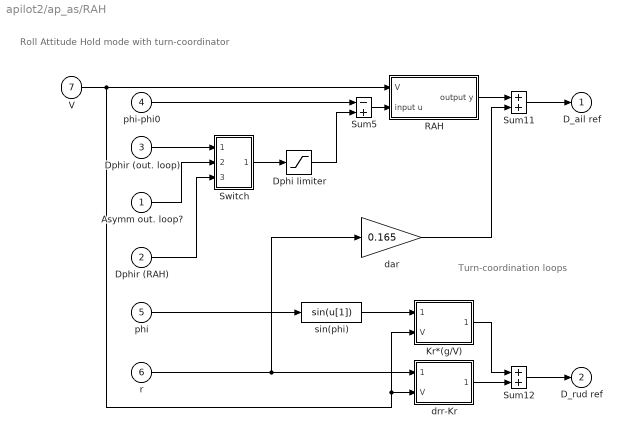
== system apilot2/ap_as/RAH ==
  note: Turn-coordination loops
  note: Roll Attitude Hold mode
      | with turn-coordinator
  Asymm out. loop? : Inport  Port=1  PortWidth=-1  SampleTime=-1
  Dphir (RAH) : Inport  Port=2  PortWidth=-1  SampleTime=-1
  Dphir (out. loop) : Inport  Port=3  PortWidth=-1  SampleTime=-1
  phi-phi0 : Inport  Port=4  PortWidth=-1  SampleTime=-1
  phi : Inport  Port=5  PortWidth=-1  SampleTime=-1
  r : Inport  Port=6  PortWidth=-1  SampleTime=-1
  V : Inport  Port=7  PortWidth=-1  SampleTime=-1
  Dphi limiter : Saturate  UpperLimit=30*pi/180  LowerLimit=-30*pi/180
  Kr*(g/V) : Subsystem
      mask Display: plot(0,0,100,100,[0,100,0],[0,50,100]);disp('K(u2)      ')
  RAH : Subsystem
      mask Display: disp('RAH (limited \n PI controller)')
  Sum11 : Sum  Inputs=++
  Sum12 : Sum  Inputs=++
  Sum5 : Sum  Inputs=-+
  Switch : Subsystem
      mask Display: plot(0,0,100,100,[100,70,40,0],[50,50,80,80],[40,0],[20,20],[29,29,0],[64,50,50],[29,29],[36,50],[40,40,41,40,39,40],[80,82,80,78,80,82],[40,40,41,40,39,40],[19,21,20,18,20,23])
  dar : Gain  Gain=0.165
  drr-Kr : Subsystem
      mask Display: plot(0,0,100,100,[0,100,0],[0,50,100]);disp('K(u2)      ')
  sin(phi) : Fcn  Expr=sin(u[1])
  D_ail ref : Outport  Port=1  InitialOutput=0
  D_rud ref : Outport  Port=2  InitialOutput=0
  wires:
  V/1 -> RAH/1(V), Kr*(g/V)/2(V), drr-Kr/2(V)
  phi/1 -> sin(phi)/1
  phi-phi0/1 -> Sum5/1
  Switch/1(Dphir) -> Dphi limiter/1
  RAH/1(output y) -> Sum11/1
  Sum11/1 -> D_ail ref/1
  Sum12/1 -> D_rud ref/1
  drr-Kr/1(y = K*u) -> Sum12/2
  sin(phi)/1 -> Kr*(g/V)/1(input u)
  Kr*(g/V)/1(y = K*u) -> Sum12/1
  dar/1 -> Sum11/2
  Sum5/1 -> RAH/2(input u)
  Dphi limiter/1 -> Sum5/2
  r/1 -> drr-Kr/1(input u), dar/1
  Dphir (out. loop)/1 -> Switch/1(Dphir (out. loop))
  Asymm out. loop?/1 -> Switch/2(Asymm.  out. loop?)
  Dphir (RAH)/1 -> Switch/3(Dphir (RAH))

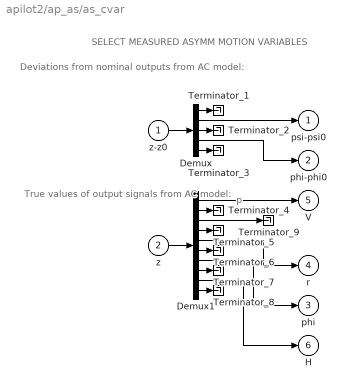
== system apilot2/ap_as/as_cvar ==
  note: p
  note: SELECT MEASURED ASYMM MOTION VARIABLES
  note: Deviations from nominal
      | outputs from AC model:
  note: True values of output
      | signals from AC model:
  z-z0 : Inport  Port=1  PortWidth=-1  SampleTime=-1
  z : Inport  Port=2  PortWidth=-1  SampleTime=-1
  Demux : Demux  Outputs=[6 1 1 1 4]
  Demux1 : Demux  Outputs=[1 2 1 1 1 2 1 2 1 1]
  Terminator_{1..9} (9 alike) : Terminator
  psi-psi0 : Outport  Port=1  InitialOutput=0
  phi-phi0 : Outport  Port=2  InitialOutput=0
  phi : Outport  Port=3  InitialOutput=0
  r : Outport  Port=4  InitialOutput=0
  V : Outport  Port=5  InitialOutput=0
  H : Outport  Port=6  InitialOutput=0
  wires:
  z-z0/1 -> Demux/1
  Demux/2 -> psi-psi0/1
  Demux/4 -> phi-phi0/1
  Demux/1 -> Terminator_1/1
  Demux/3 -> Terminator_2/1
  Demux/5 -> Terminator_3/1
  Demux1/9 -> H/1
  z/1 -> Demux1/1
  Demux1/3 -> Terminator_9/1
  Demux1/5 -> r/1
  Demux1/7 -> phi/1
  Demux1/2 -> Terminator_4/1
  Demux1/4 -> Terminator_5/1
  Demux1/6 -> Terminator_6/1
  Demux1/8 -> Terminator_7/1
  Demux1/10 -> Terminator_8/1
  Demux1/1 -> V/1

== system apilot2/ap_as/as_mc ==
  note: SELECT ASYMM MODE (on/off flags denoted by '?')
  note: SELECT ASYMM REFERENCE SIGNALS
  ymode : Inport  Port=1  PortWidth=-1  SampleTime=-1
  yref : Inport  Port=2  PortWidth=-1  SampleTime=-1
  Demux : Demux  Outputs=[5 1 1 1 1 1]
  Demux1 : Demux  Outputs=[3 1 1]
  Terminator_1 : Terminator
  Terminator_2 : Terminator
  asymm. mode? : Outport  Port=1  InitialOutput=0
  asymm. out. loop? : Outport  Port=2  InitialOutput=0
  Dphir (RAH) : Outport  Port=3  InitialOutput=0
  HH? : Outport  Port=4  InitialOutput=0
  Dpsir (HH) : Outport  Port=5  InitialOutput=0
  NAV? : Outport  Port=6  InitialOutput=0
  LOC coupled? : Outport  Port=7  InitialOutput=0
  wires:
  yref/1 -> Demux1/1
  Demux1/2 -> Dphir (RAH)/1
  Demux1/3 -> Dpsir (HH)/1
  ymode/1 -> Demux/1
  Demux/2 -> asymm. mode?/1
  Demux/3 -> asymm. out. loop?/1
  Demux/4 -> HH?/1
  Demux/5 -> NAV?/1
  Demux/6 -> LOC coupled?/1
  Demux/1 -> Terminator_1/1
  Demux1/1 -> Terminator_2/1

== system apilot2/ap_as/t ==

== system apilot2/ap_s/1/Ktheta ==
  input u : Inport  Port=1  PortWidth=-1  SampleTime=-1
  V : Inport  Port=2  PortWidth=-1  SampleTime=-1
  1/Ktheta : Fcn  Expr=1/(-1.375*10^(-3)*u[1]^2 + 0.1575*u[1] - 4.8031)
  Product : Product  Inputs=2
  y = K*u : Outport  Port=1  InitialOutput=0
  wires:
  V/1 -> 1/Ktheta/1
  Product/1 -> y = K*u/1
  input u/1 -> Product/2
  1/Ktheta/1 -> Product/1

== system apilot2/ap_s/ALH ==
  note: Altitude Hold mode
  ALH? : Inport  Port=1  PortWidth=-1  SampleTime=-1
  DHr (ALH) : Inport  Port=2  PortWidth=-1  SampleTime=-1
  H-H0 : Inport  Port=3  PortWidth=-1  SampleTime=-1
  V : Inport  Port=4  PortWidth=-1  SampleTime=-1
  KH : Subsystem
      mask Display: plot(0,0,100,100,[0,100,0],[0,50,100]);disp('K(u1)      ')
  On/Off : Subsystem
      mask Type: On/off switch
      mask Description:
      | If input(1) = 1
      |      output = input(2)
      |  else if input(1) = 0
      |      output = 0
      mask Help: On/off switch.
      mask Display: plot(0,0,100,100,[31,31,32,34,34,32,31,31,0],[50,48,47,48,51,53,51,50,50],[100,75,51],[50,50,97]);disp('?')
  Sum : Sum  Inputs=+-
  Dthetar (ALH) : Outport  Port=1  InitialOutput=0
  wires:
  V/1 -> KH/1(V)
  Sum/1 -> KH/2(input u)
  KH/1(y = K*u) -> On/Off/2(in)
  ALH?/1 -> On/Off/1(crit)
  DHr (ALH)/1 -> Sum/1
  On/Off/1(out) -> Dthetar (ALH)/1
  H-H0/1 -> Sum/2

== system apilot2/ap_s/ALS ==
  note: Altitude Select Mode
  ALS? : Inport  Port=1  PortWidth=-1  SampleTime=-1
  DHdot r (ALS) : Inport  Port=2  PortWidth=-1  SampleTime=-1
  Hdot-Hdot0 : Inport  Port=3  PortWidth=-1  SampleTime=-1
  V : Inport  Port=4  PortWidth=-1  SampleTime=-1
  KHdot : Subsystem
      mask Display: plot(0,0,100,100,[0,100,0],[0,50,100]);disp('K(u1)      ')
  On/Off : Subsystem
      mask Type: On/off switch
      mask Description:
      | If input(1) = 1
      |      output = input(2)
      |  else if input(1) = 0
      |      output = 0
      mask Help: On/off switch.
      mask Display: plot(0,0,100,100,[31,31,32,34,34,32,31,31,0],[50,48,47,48,51,53,51,50,50],[100,75,51],[50,50,97]);disp('?')
  Sum : Sum  Inputs=+-
  filter : TransferFcn  Numerator=[1]  Denominator=[1 0.15]
  Dthetar (ALS) : Outport  Port=1  InitialOutput=0
  wires:
  V/1 -> KHdot/1(V)
  Hdot-Hdot0/1 -> Sum/2
  KHdot/1(y = K*u) -> On/Off/2(in)
  ALS?/1 -> On/Off/1(crit)
  DHdot r (ALS)/1 -> Sum/1
  On/Off/1(out) -> Dthetar (ALS)/1
  Sum/1 -> filter/1
  filter/1 -> KHdot/2(input u)

== system apilot2/ap_s/GS ==
  note: Glideslope coupled mode
  GS coupled? : Inport  Port=1  PortWidth=-1  SampleTime=-1
  epsilon_gs : Inport  Port=2  PortWidth=-1  SampleTime=-1
  d(epsilon_gs)/dt : Inport  Port=3  PortWidth=-1  SampleTime=-1
  V : Inport  Port=4  PortWidth=-1  SampleTime=-1
  H : Inport  Port=5  PortWidth=-1  SampleTime=-1
  Keps_gs : Subsystem
      mask Display: plot(0,0,100,100,[0,100,0],[0,50,100]);disp('K(u1)      ')
  Kr : Gain  Gain=1
  On/Off : Subsystem
      mask Type: On/off switch
      mask Description:
      | If input(1) = 1
      |      output = input(2)
      |  else if input(1) = 0
      |      output = 0
      mask Help: On/off switch.
      mask Display: plot(0,0,100,100,[31,31,32,34,34,32,31,31,0],[50,48,47,48,51,53,51,50,50],[100,75,51],[50,50,97]);disp('?')
  Rgs approximation : Fcn  Expr=(u[1]-HRW)/sin(abs(gamgs*pi/180)) + xgs
  Sum : Sum  Inputs=++
  prod : Product  Inputs=2
  Dthetar (GS) : Outport  Port=1  InitialOutput=0
  wires:
  On/Off/1(out) -> Dthetar (GS)/1
  Keps_gs/1(y = K*u) -> On/Off/2(in)
  prod/1 -> Keps_gs/2(input u)
  Rgs approximation/1 -> prod/2
  Sum/1 -> prod/1
  Kr/1 -> Sum/2
  d(epsilon_gs)/dt/1 -> Kr/1
  epsilon_gs/1 -> Sum/1
  V/1 -> Keps_gs/1(V)
  GS coupled?/1 -> On/Off/1(crit)
  H/1 -> Rgs approximation/1

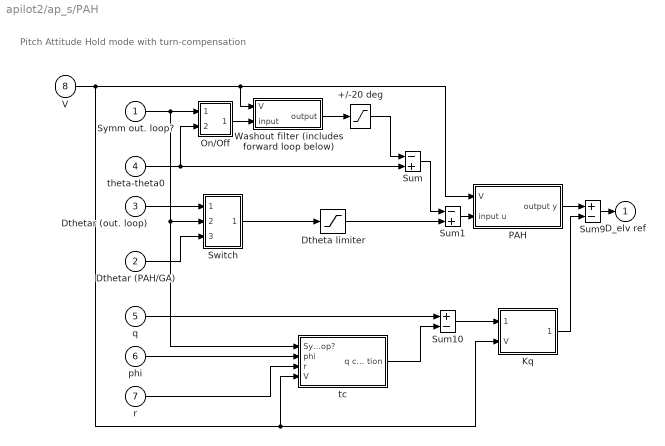
== system apilot2/ap_s/PAH ==
  note: Pitch Attitude Hold mode
      | with turn-compensation
  Symm out. loop? : Inport  Port=1  PortWidth=-1  SampleTime=-1
  Dthetar (PAH/GA) : Inport  Port=2  PortWidth=-1  SampleTime=-1
  Dthetar (out. loop) : Inport  Port=3  PortWidth=-1  SampleTime=-1
  theta-theta0 : Inport  Port=4  PortWidth=-1  SampleTime=-1
  q : Inport  Port=5  PortWidth=-1  SampleTime=-1
  phi : Inport  Port=6  PortWidth=-1  SampleTime=-1
  r : Inport  Port=7  PortWidth=-1  SampleTime=-1
  V : Inport  Port=8  PortWidth=-1  SampleTime=-1
  +/-20 deg : Saturate  UpperLimit=20*(pi/180)  LowerLimit=-20*(pi/180)
  Dtheta limiter : Saturate  UpperLimit=18*(pi/180)  LowerLimit=-8*(pi/180)
  Kq : Subsystem
      mask Display: plot(0,0,100,100,[0,100,0],[0,50,100]);disp('K(u2)      ')
  On/Off : Subsystem
      mask Type: On/off switch
      mask Description:
      | If input(1) = 1
      |      output = input(2)
      |  else if input(1) = 0
      |      output = 0
      mask Help: On/off switch. \nIf input(1) = 1, the output equals input(2). \nIf input(1) = 0, the output is zero.
      mask Display: plot(0,0,100,100,[31,31,32,34,34,32,31,31,0],[50,48,47,48,51,53,51,50,50],[100,75,51],[50,50,97]);disp('?')
  PAH : Subsystem
      mask Display: disp('PAH (limited \n PI controller)')
  Sum : Sum  Inputs=-+
  Sum1 : Sum  Inputs=-+
  Sum10 : Sum  Inputs=+-
  Sum9 : Sum  Inputs=+-
  Switch : Subsystem
      mask Display: plot(0,0,100,100,[100,70,40,0],[50,50,80,80],[40,0],[20,20],[29,29,0],[64,50,50],[29,29],[36,50],[40,40,41,40,39,40],[80,82,80,78,80,82],[40,40,41,40,39,40],[19,21,20,18,20,23])
  Washout filter (includes forward loop below) : Subsystem
      mask Display: disp('Kd/(s+Kd)')
  tc : Subsystem
      mask Display: disp('Turn\nCompensator')
  D_elv ref : Outport  Port=1  InitialOutput=0
  wires:
  Symm out. loop?/1 -> On/Off/1(crit.), tc/1(Symm. outer loop?), Switch/2(Symm.  out. loop?)
  Dthetar (out. loop)/1 -> Switch/1(Dthetar (out. loop))
  Switch/1(Dthetar) -> Dtheta limiter/1
  r/1 -> tc/3(r)
  phi/1 -> tc/2(phi)
  Washout filter (includes forward loop below)/1(output) -> +/-20 deg/1
  On/Off/1(out) -> Washout filter (includes forward loop below)/2(input)
  Sum9/1 -> D_elv ref/1
  Sum1/1 -> PAH/2(input u)
  Dtheta limiter/1 -> Sum1/2
  PAH/1(output y) -> Sum9/1
  Sum10/1 -> Kq/1(input u)
  q/1 -> Sum10/1
  Kq/1(y = K*u) -> Sum9/2
  V/1 -> Kq/2(V), tc/4(V), PAH/1(V), Washout filter (includes forward loop below)/1(V)
  tc/1(q correc- tion) -> Sum10/2
  Sum/1 -> Sum1/1
  +/-20 deg/1 -> Sum/1
  theta-theta0/1 -> Sum/2, On/Off/2(in)
  Dthetar (PAH/GA)/1 -> Switch/3(Dthetar (PAH/RAH))

== system apilot2/ap_s/Symm. mode On/Off ==
  crit : Inport  Port=1  PortWidth=-1  SampleTime=-1
  in : Inport  Port=2  PortWidth=-1  SampleTime=-1
  Sum : Sum  Inputs=+-
  Switch : Switch  Threshold=0
  const. : Constant  Value=0.5
  const.1 : Constant  Value=0
  out : Outport  Port=1  InitialOutput=0
  wires:
  crit/1 -> Sum/1
  const.1/1 -> Switch/3
  Sum/1 -> Switch/2
  Switch/1 -> out/1
  in/1 -> Switch/1
  const./1 -> Sum/2

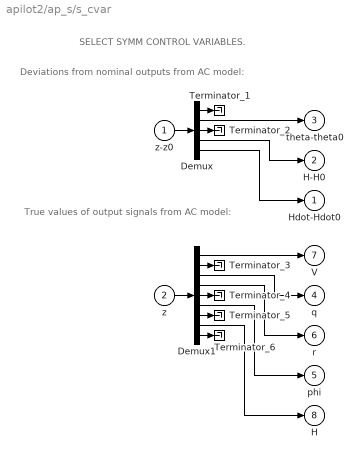
== system apilot2/ap_s/s_cvar ==
  note: SELECT SYMM CONTROL VARIABLES.
  note: True values of output
      | signals from AC model:
  note: Deviations from nominal
      | outputs from AC model:
  z-z0 : Inport  Port=1  PortWidth=-1  SampleTime=-1
  z : Inport  Port=2  PortWidth=-1  SampleTime=-1
  Demux : Demux  Outputs=[7 1 3 1 1]
  Demux1 : Demux  Outputs=[1 3 1 1 2 1 2 1 1]
  Terminator_{1..6} (6 alike) : Terminator
  Hdot-Hdot0 : Outport  Port=1  InitialOutput=0
  H-H0 : Outport  Port=2  InitialOutput=0
  theta-theta0 : Outport  Port=3  InitialOutput=0
  q : Outport  Port=4  InitialOutput=0
  phi : Outport  Port=5  InitialOutput=0
  r : Outport  Port=6  InitialOutput=0
  V : Outport  Port=7  InitialOutput=0
  H : Outport  Port=8  InitialOutput=0
  wires:
  z/1 -> Demux1/1
  Demux1/2 -> Terminator_3/1
  Demux1/5 -> Terminator_4/1
  Demux1/7 -> Terminator_5/1
  Demux1/9 -> Terminator_6/1
  Demux1/1 -> V/1
  Demux1/3 -> q/1
  Demux1/4 -> r/1
  Demux1/6 -> phi/1
  Demux1/8 -> H/1
  z-z0/1 -> Demux/1
  Demux/1 -> Terminator_1/1
  Demux/3 -> Terminator_2/1
  Demux/5 -> Hdot-Hdot0/1
  Demux/4 -> H-H0/1
  Demux/2 -> theta-theta0/1

== system apilot2/ap_s/s_mc ==
  note: SELECT SYMM MODE (on/off flags denoted by '?')
  note: SELECT SYMM REFERENCE SIGNALS
  ymode : Inport  Port=1  PortWidth=-1  SampleTime=-1
  yref : Inport  Port=2  PortWidth=-1  SampleTime=-1
  Demux : Demux  Outputs=[1 1 1 1 1 5]
  Demux1 : Demux  Outputs=[1 1 1 2]
  Terminator_1 : Terminator
  Terminator_2 : Terminator
  symm mode? : Outport  Port=1  InitialOutput=0
  symm. outer loop? : Outport  Port=2  InitialOutput=0
  Dthetar (PAH) : Outport  Port=3  InitialOutput=0
  ALS? : Outport  Port=4  InitialOutput=0
  DHdot r (ALS) : Outport  Port=5  InitialOutput=0
  ALH? : Outport  Port=6  InitialOutput=0
  DHr (ALH) : Outport  Port=7  InitialOutput=0
  GS coupled? : Outport  Port=8  InitialOutput=0
  wires:
  Demux1/3 -> DHdot r (ALS)/1
  Demux1/2 -> DHr (ALH)/1
  Demux1/1 -> Dthetar (PAH)/1
  Demux/5 -> GS coupled?/1
  Demux/4 -> ALS?/1
  Demux/3 -> ALH?/1
  Demux/1 -> symm mode?/1
  Demux/2 -> symm. outer loop?/1
  yref/1 -> Demux1/1
  Demux1/4 -> Terminator_2/1
  ymode/1 -> Demux/1
  Demux/6 -> Terminator_1/1

== system apilot2/ap_s/t ==

== system apilot2/d+l/t ==

== system apilot2/Beaver dynamics/AC/0 ==

== system apilot2/Beaver dynamics/AC/ad ==
  x : Inport  Port=1  PortWidth=-1  SampleTime=-1
  0 : Subsystem
      settings: OpenFcn=fdchelp adgrp
      mask Display: disp('AIRDATA GROUP (level 3)\nM.O. Rauw')
  ad1 : Subsystem
      mask Type: Airdata1
      mask Description: Basic airdata variables
      mask Help: eval('fdchelp airdata1')
      mask Display: disp('Airdata1')
  ad2 : Subsystem
      mask Type: Airdata2
      mask Description: More airdata variables
      mask Help: eval('fdchelp airdata2')
      mask Display: disp('Airdata2')
  ad3 : Subsystem  mask(Airdata3){cbar=GM1(1)}
      mask prompts: cbar "Mean aerodynamic chord [m]:"
      mask help: More airdata variables
      mask Help: eval('fdchelp airdata3')
      mask Display: disp('Airdata3')
  atm : Subsystem
      mask Type: Atmosph
      mask Description: Atmosphere variables
      mask Help: eval('fdchelp atmosph')
      mask Display: disp('Atmosph')
  yatm : Outport  Port=1  InitialOutput=0
  yad1 : Outport  Port=2  InitialOutput=0
  yad2 : Outport  Port=3  InitialOutput=0
  yad3 : Outport  Port=4  InitialOutput=0
  wires:
  ad1/1(yad1) -> ad3/3(yad1), ad2/2(yad1), yad1/1
  atm/1(yatm) -> ad3/2(yatm), ad2/1(yatm), ad1/2(yatm), yatm/1
  x/1 -> ad3/1(x), ad1/1(x), atm/1(x)
  ad3/1(yad3) -> yad3/1
  ad2/1(yad2) -> yad2/1

== system apilot2/Beaver dynamics/AC/ae ==
  x : Inport  Port=1  PortWidth=-1  SampleTime=-1
  uaero : Inport  Port=2  PortWidth=-1  SampleTime=-1
  yad1 : Inport  Port=3  PortWidth=-1  SampleTime=-1
  0 : Subsystem
      settings: OpenFcn=fdchelp aerogrp
      mask Display: disp('AERODYNAMICS GROUP (level 3)\nM.O. Rauw')
  aero : Subsystem
      mask Type: Aeromod
      mask Description: Aerodynamic model of the DHC-2 'Beaver'.
      mask Help: eval('fdchelp aeromod')
      mask Display: disp('Aeromod\n(Beaver)')
  dl : Subsystem  mask(Dimless){cbar=GM1(1), b=GM1(2)}
      mask prompts: cbar "Mean aerodynamic chord [m]:"; b "Wing span [m]:"
      mask help: Dimensionless rotational velocities.
      mask Help: eval('fdchelp dimless')
      mask Display: disp('Dimless')
  fmdims : Subsystem  mask(FMdims){cbar=GM1(1), b=GM1(2), S=GM1(3)}
      mask prompts: cbar "Mean aerodynamic chord [m]:"; b "Wing span [m]:"; S "Wing surface [m^2]:"
      mask help:
      | Calculate forces and moments from
      | dimensionless coefficients.
      mask Help: eval('fdchelp fmdims')
      mask Display: disp('FMdims')
  ydl : Outport  Port=1  InitialOutput=0
  Caero : Outport  Port=2  InitialOutput=0
  FMaero : Outport  Port=3  InitialOutput=0
  wires:
  fmdims/1(Forces and moments) -> FMaero/1
  yad1/1 -> fmdims/1(yad1)
  uaero/1 -> aero/2(uaero)
  x/1 -> aero/1(x), dl/1(x)
  dl/1(ydl) -> aero/3(ydl), ydl/1
  aero/1(Caero) -> fmdims/2(Force / moment coefficients), Caero/1

== system apilot2/Beaver dynamics/AC/eng ==
  x : Inport  Port=1  PortWidth=-1  SampleTime=-1
  uprop : Inport  Port=2  PortWidth=-1  SampleTime=-1
  yatm : Inport  Port=3  PortWidth=-1  SampleTime=-1
  yad1 : Inport  Port=4  PortWidth=-1  SampleTime=-1
  0 : Subsystem
      settings: OpenFcn=fdchelp enggrp
      mask Display: disp('ENGINE GROUP (level 3)\nM.O. Rauw')
  eng : Subsystem
      mask Type: Engmod
      mask Description: Engine model for the DHC-2 'Beaver'
      mask Help: eval('fdchelp engmod')
      mask Display: disp('Engmod\n(Beaver)')
  fmdims : Subsystem  mask(FMdims){cbar=GM1(1), b=GM1(2), S=GM1(3)}
      mask prompts: cbar "Mean aerodynamic chord [m]:"; b "Wing span [m]:"; S "Wing surface [m^2]:"
      mask help:
      | Calculate forces and moments from
      | dimensionless coefficients.
      mask Help: eval('fdchelp fmdims')
      mask Display: disp('FMdims')
  pow : Subsystem
      mask Type: Power
      mask Description:
      | Engine power and dimensionless
      | pressure increase across propeller
      | (model for DHC-2 'Beaver')
      mask Help: eval('fdchelp power')
      mask Display: disp('Power\n(Beaver)')
  ypow : Outport  Port=1  InitialOutput=0
  Cprop : Outport  Port=2  InitialOutput=0
  FMprop : Outport  Port=3  InitialOutput=0
  wires:
  yatm/1 -> pow/3(yatm)
  x/1 -> eng/1(x), pow/1(x)
  yad1/1 -> fmdims/1(yad1)
  eng/1(Cprop) -> fmdims/2(Force / moment coefficients), Cprop/1
  fmdims/1(Forces and moments) -> FMprop/1
  uprop/1 -> pow/2(uprop)
  pow/1(ypow) -> eng/2(ypow), ypow/1

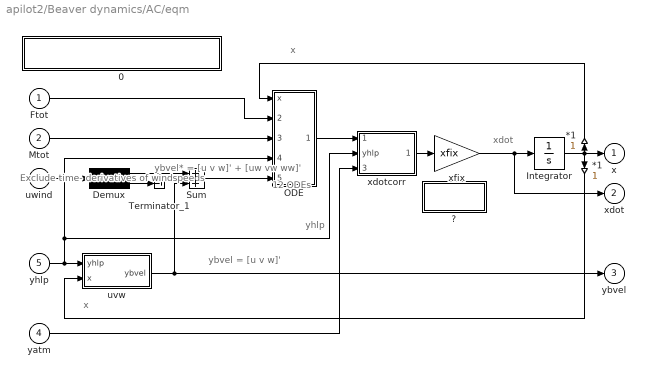
== system apilot2/Beaver dynamics/AC/eqm ==
  note: 12 ODEs
  note: ybvel = [u v w]'
  note: yhlp
  note: x
  note: x
  note: xdot
  note: ybvel* =
      | [u v w]' +
      | [uw vw ww]'
  note: Exclude time-
      | derivatives
      | of windspeeds
  Ftot : Inport  Port=1  PortWidth=-1  SampleTime=-1
  Mtot : Inport  Port=2  PortWidth=-1  SampleTime=-1
  uwind : Inport  Port=3  PortWidth=-1  SampleTime=-1
  yatm : Inport  Port=4  PortWidth=-1  SampleTime=-1
  yhlp : Inport  Port=5  PortWidth=-1  SampleTime=-1
  " *1" : Gain  Orientation=up  Gain=1
  *1 : Gain  Orientation=down  Gain=1
  0 : Subsystem
      settings: OpenFcn=fdchelp eqmotion
      mask Display: disp('EQUATIONS OF MOTION (level 3)\nM.O. Rauw')
  "?" : Subsystem
      settings: OpenFcn=fdchelp xfix
      mask Display: disp('More info\nfor xfix')
  Demux : Demux  Outputs=[3 3]
  Integrator : Integrator  ExternalReset=none  InitialConditionSource=internal  InitialCondition=xinco  LimitOutput=off  UpperSaturationLimit=inf  LowerSaturationLimit=-inf  ShowSaturationPort=off  ShowStatePort=off  AbsoluteTolerance=auto
  ODE : Subsystem
  Sum : Sum  Inputs=++
  Terminator_1 : Terminator
  uvw : Subsystem
      mask Type: uvw
      mask Description:
      | Calculation of body-axes velocities
      | u, v, and w
      mask Help: eval('fdchelp uvw')
      mask Display: disp('Body-axes\nvelocities')
  xdotcorr : Subsystem  mask(xdotcorr){b=GM1(2), S=GM1(3), m=GM1(10), CYbdot=AM(2,19)}
      mask prompts: b "Wing span [m]:"; S "Wing surface [m^2]:"; m "Mass of the aircraft [kg]:"; CYbdot "Stability-derivative CYbdot:"
      mask help:
      | Correction block to write state
      | equations for DHC-2 Beaver aircraft
      | explicitly.
      mask Help: eval('fdchelp xdotcorr')
      mask Display: disp('xdotcorr\n(Beaver)')
  xfix : Gain  Gain=xfix
  x : Outport  Port=1  InitialOutput=0
  xdot : Outport  Port=2  InitialOutput=0
  ybvel : Outport  Port=3  InitialOutput=0
  wires:
  " *1"/1 -> ODE/1(x)
  xfix/1 -> xdot/1, Integrator/1
  Integrator/1 -> *1/1, " *1"/1, x/1
  *1/1 -> uvw/2(x)
  Mtot/1 -> ODE/3(Mtot)
  Ftot/1 -> ODE/2(Ftot)
  yatm/1 -> xdotcorr/3(yatm)
  xdotcorr/1(xdot corrected) -> xfix/1
  Demux/1 -> Sum/1
  uwind/1 -> Demux/1
  uvw/1(ybvel) -> Sum/2, ybvel/1
  Sum/1 -> ODE/5(ybvel*)
  ODE/1(xdot) -> xdotcorr/1(xdot uncorrected)
  yhlp/1 -> xdotcorr/2(yhlp), ODE/4(yhlp), uvw/1(yhlp)
  Demux/2 -> Terminator_1/1
